simulink model "ep10_24"  (R2018a)
settings: Solver=VariableStepAuto  StartTime=0.0  StopTime=30  MaxStep=0.001  RelTol=1e-3
settings Model: Creator=zheny  LastModifiedBy=zheny

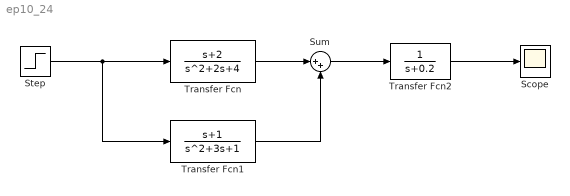
== system ep10_24 ==
  Scope : Scope
  Step : Step  SampleTime=0
  Sum : Sum  Inputs=|++
  Transfer Fcn : TransferFcn  Numerator=[1 2]  Denominator=[1 2 4]
  Transfer Fcn1 : TransferFcn  Numerator=[1 1]  Denominator=[1 3 1]
  Transfer Fcn2 : TransferFcn  Denominator=[1 0.2]
  wires:
  Transfer Fcn/1 -> Sum/1
  Sum/1 -> Transfer Fcn2/1
  Transfer Fcn1/1 -> Sum/2
  Step/1 -> Transfer Fcn1/1, Transfer Fcn/1
  Transfer Fcn2/1 -> Scope/1
